simulink model "menabport_noio"  (Simulink 8.0)
settings: Solver=FixedStepDiscrete  StartTime=0.0  StopTime=10.0  FixedStep=1  RelTol=1e-3
settings Model: Creator=mtocci  LastModifiedBy=mtocci
settings DataIOCC: LimitDataPoints=off  SaveFormat=StructureWithTime  SignalLoggingSaveFormat=ModelDataLogs
settings OptimizationCC: InlineParams=on
settings DebuggingCC: FcnCallInpInsideContextMsg=Use local settings  StrictBusMsg=ErrorOnBusTreatedAsVector
settings GRTTargetCC: CombineOutputUpdateFcns=off

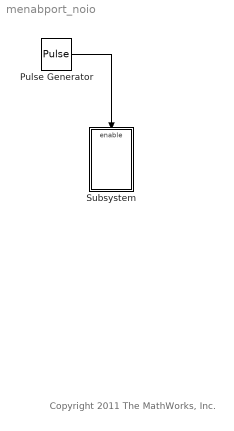
== system menabport_noio ==
  note: Copyright 2011 The MathWorks, Inc.
  Pulse Generator : DiscretePulseGenerator  Amplitude=[1 1 2 2]
  Subsystem : Subsystem
  wires:
  Pulse Generator/1 -> Subsystem/Enable

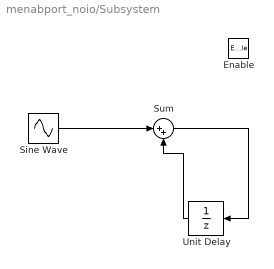
== system menabport_noio/Subsystem ==
  Enable : EnablePort
  Sine Wave : Sin  SineType=Sample based  Samples=5  SampleTime=1
  Sum : Sum  Inputs=|++
  Unit Delay : UnitDelay  SampleTime=-1
  wires:
  Sum/1 -> Unit Delay/1
  Unit Delay/1 -> Sum/2
  Sine Wave/1 -> Sum/1
